simulink model "SimulationANTSMC"  (R2020b)
(part 15 of 18)

                                                                                                                                                                                                                                                                                                                                                                                                                                                                                                                                                                                                                                                                                                                                                                                                                                                                                                                                                                                                                                                                                                                                                                                                                                                                                                                                                                                                                                                                                                                                                                                                                                                                                                                                                                                                                                                                                                                                                                                                                                                                                                                                                                                                                                                                                                                                                                                                                                                                                                                                                                                                                                                                                                                                                                                                                                                                                                                                                                                                                                                                                                                                                                                                                                                                                                                                                                                                                                                                                                                                                                                                                                                                                                                                                                                                                                                                                                                                                                                                                                                                                                                                                                                                                                                                                                                                                                                                                                                                                                                                                                                                                                                                                                                                                                                                                                                                                                                                                                                                                                                                                                                                                                                                                                                                                                                                                                                                                                                                                                                                                                                                                                                                                                                                                                                                                                                                                                                                                                                                                                                                                                                                                                                                                                                                                                                                                                                                                                                                                                                                                                                                                                                                                                                                                                                                                                                                                                                                                                                                                                                                                                                                                                                                                                                                                                                                                                                                                                                                                                                                                                                                                                                                                                                                                                                                                                                                                                                                                                                                                                                                                                                                                                                                                                                                                                                                                                                                                                                                                                                                                                                                                                                                                                                                                                                                                                                                                                                                                                                                                                                                                                                                                                                                                                                                                                                                                                                                                                                                                                                                                                                                                                                                                                                                                                                                                                                                                                                                                                                                                                                                                                                                                                                                                                                                                                                                                                                                                                                                                                                                                                                                                                                                                                                                                                                                                                                                                                                                                                                                                                                                                                                                                                                                                                                                                                                                                                                                                                                                                                                                                                                                                                                                                                                                                                                                                                                                                                                                                                                                                                                                                                                                                                                                                                                                                                                                                                                                                                                                                                                                                                                                                                                                                                                                                                                                                                                                                                                                                                                                                                                                                                                                                                                                                                                                                                                                                                                                                                                                                                                                                                                                                                                                                                                                                                                                                                                                                                                                                                                                                                                                                                                                                                                                                                                                                                                                                                                                                                                                                                                                                                                                                                                                                                                                                                                                                                                                                                                                                                                                                                                                                                                                                                                                                                                                                                                                                                                                                                                                                                                                                                                                                                                                                                                                                                                                                                                                                                                                                                                                                                                                                                                                                                                                                                                                                                                                                                                                                                                                                                                                                                                                                                                                                                                                                                                                                                                                                                                                                                                                                                                                                                                                                                                                                                                                                                                                                                                                                                                                                                                                                                                                                                                                                                                                                                                                                                                                                                                                                                                                                                                                                                                                                                                                                                                                                                                                                                                                                                                                                                                                                                                                                                                                                                                                                                                                                                                                                                                                                                                                                                                                                                                                                                                                                                                                                                                                                                                                                                                                                                                                                                                                                                                                                                                                                                                                                                                                                                                                                                                                                                                                                                                                                                                                                                                                                                                                                                                                                                                                                                                                                                                                                                                                                                                                                                                                                                                                                                                                                                                                                                                                                                                                                                                                                                                                                                                                                                                                                                                                                                                                                                                                                                                                                                                                                                                                                                                                                                                                                                                                                                                                                                                                                                                                                                                                                                                                                                                                                                                                                                                                                                                                                                                                                                                                                                                                                                                                                                                                                                                                                                                                                                                                                                                                                                                                                                                                                                                                                                                                                                                                                                                                                                                                                                                                                                                                                                                                                                                                                                                                                                                                                                                                                                                                                                                                                                                                                                                                                                                                                                                                                                                                                                                                                                                                                                                                                                                                                                                                                                                                                                                                                                                                                                                                                                                                                                                                                                                                                                                                                                                                                                                                                                                                                                                                                                                                                                                                                                                                                                                                                                                                                                                                                                                                                                                                                                                                                                                                                                                                                                                                                                                                                                                                                                                                                                                                                                                                                                                                                                                                                                                                                                                                                                                                                                                                                                                                                                                                                                                                                                                                                                                                                                                                                                                                                                                                                                                                                                                                                                                                                                                                                                                                                                                                                                                                                                                                                                                                                                                                                                                                                                                                                                                                                                                                                                                                                                                                                                                                                                                                                                                                                                                                                                                                                                                                                                                                                                                                                                                                                                                                                                                                                                                                                                                                                                                                                                                                                                                                                                                                                                                                                                                                                                                                                                                                                                                                                                                                                                                                                                                                                                                                                                                                                                                                                                                                                                                                                                                                                                                                                                                                                                                                                                                                                                                                                                                                                                                                                                                                                                                                                                                                                                                                                                                                                                                                                                                                                                                                                                                                                                                                                                                                                                                                                                                                                                                                                                                                                                                                                                                                                                                                                                                                                                                                                                                                                                                                                                                                                                                                                                                                                                                                                                                                                                                                                                                                                                                                                                                                                                                                                                                                                                                                                                                                                                                                                                                                                                                                                                                                                                                                                                                                                                                                                                                                                                                                                                                                                                                                                                                                                                                                                                                                                                                                                                                                                                                                                                                                                                                                                                                                                                                                                                                                                                                                                                                                                                                                                                                                                                                                                                                                                                                                                                                                                                                                                                                                                                                                                                                                                                                                                                                                                                                                                                                                                                                                                                                                                                                                                                                                                                                                                                                                                                                                                                                                                                                                                                                                                                                                                                                                                                                                                                                                                                                                                                                                                                                                                                                                                                                                                                                                                                                                                                                                                                                                                                                                                                                                                                                                                                                                                                                                                                                                                                                                                                                                                                                                                                                                                                                                                                                                                                                                                                                                                                                                                                                                                                                                                                                                                                                                                                                                                                                                                                                                                                                                                                                                                                                                                                                                                                                                                                                                                                                                                                                                                                                                                                                                                                                                                                                                                                                                                                                                                                                                                                                                                                                                                                                                                                                                                                                                                                                                                                                                                                                                                                                                                                                                                                                                                                                                                                                                                                                                                                                                                                                                                                                                                                                                                                                                                                                                                                                                                                                                                                                                                                                                                                                                                                                                                                                                                                                                                                                                                                                                                                                                                                                                                                                                                                                                                                                                                                                                                                                                                                                                                                                                                                                                                                                                                                                                                                                                                                                                                                                                                                                                                                                                                                                                                                                                                                                                                                                                                                                                                                                                                                                                                                                                                                                                                                                                                                                                                                                                                                                                                                                                                                                                                                                                                                                                                                                                                                                                                                                                                                                                                                                                                                                                                                                                                                                                                                                                                                                                                                                                                                                                                                                                                                                                                                                                                                                                                                                                                                                                                                                                                                                                                                                                                                                                                                                                                                                                                                                                                                                                                                                                                                                                                                                                                                                                                                                                                                                                                                                                                                                                                                                                                                                                                                                                                                                                                                                                                                                                                                                                                                                                                                                                                                                                                                                                                                                                                                                                                                                                                                                                                                                                                                                                                                                                                                                                                                                                                                                                                                                                                                                                                                                                                                                                                                                                                                                                                                                                                                                                                                                                                                                                                                                                                                                                                                                                                                                                                                                                                                                                                                                                                                                                                                                                                                                                                                                                                                                                                                                                                                                                                                                                                                                                                                                                                                                                                                                                                                                                                                                                                                                                                                                                                                                                                                                                                                                                                                                                                                                                                                                                                                                                                                                                                                                                                                                                                                                                                                                                                                                                                                                                                                                                                                                                                                                                                                                                                                                                                                                                                                                                                                                                                                                                                                                                                                                                                                                                                                                                                                                                                                                                                                                                                                                                                                                                                                                                                                                                                                                                                                                                                                                                                                                                                                                                                                                                                                                                                                                                                                                                                                                                                                                                                                                                                                                                                                                                                                                                                                                                                                                                                                                                                                                                                                                                                                                                                                                                                                                                                                                                                                                                                                                                                                                                                                                                                                                                                                                                                                                                                                                                                                                                                                                                                                                                                                                                                                                                                                                                                                                                                                                                                                                                                                                                                                                                                                                                                                                                                                                                                                                                                                                                                                                                                                                                                                                                                                                                                                                                                                                                                                                                                                                                                                                                                                                                                                                                                                                                                                                                                                                                                                                                                                                                                                                                                                                                                                                                                                                                                                                                                                                                                                                                                                                                                                                                                                                                                                                                                                                                                                                                                                                                                                                                                                                                                                                                                                                                                                                                                                                                                                                                                                                                                                                                                                                                                                                                                                                                                                                                                                                                                                                                                                                                                                                                                                                                                                                                                                                                                                                                                                                                                                                                                                                                                                                                                                                                                                                                                                                                                                                                                                                                                                                                                                                                                                                                                                                                                                                                                                                                                                                                                                                                                                                                                                                                                                                                                                                                                                                                                                                                                                                                                                                                                                                                                                                                                                                                                                                                                                                                                                                                                                                                                                                                                                                                                                                                                                                                                                                                                                                                                                                                                                                                                                                                                                                                                                                                                                                                                                                                                                                                                                                                                                                                                                                                                                                                                                                                                                                                                                                                                                                                                                                                                                                                                                                                                                                                                                                                                                                                                                                                                                                                                                                                                                                                                                                                                                                                                                                                                                                                                                                                                                                                                                                                                                                                                                                                                                                                                                                                                                                                                                                                                                                                                                                                                                                                                                                                                                                                                                                                                                                                                                                                                                                                                                                                                                                                                                                                                                                                                                                                                                                                                                                                                                                                                                                                                                                                                                                                                                                                                                                                                                                                                                                                                                                                                                                                                                                                                                                                                                                                                                                                                                                                                                                                                                                                                                                                                                                                                                                                                                                                                                                                                                                                                                                                                                                                                                                                                                                                                                                                                                                                                                                                                                                                                                                                                                                                                                                                                                                                                                                                                                                                                                                                                                                                                                                                                                                                                                                                                                                                                                                                                                                                                                                                                                                                                                                                                                                                                                                                                                                                                                                                                                                                                                                                                                                                                                                                                                                                                                                                                                                                                                                                                                                                                                                                                                                                                                                                                                                                                                                                                                                                                                                                                                                                                                                                                                                                                                                                                                                                                                                                                                                                                                                                                                                                                                                                                                                                                                                                                                                                                                                                                                                                                                                                                                                                                                                                                                                                                                                                                                                                                                                                                                                                                                                                                                                                                                                                                                                                                                                                                                                                                                                                                                                                                                                                                                                                                                                                                                                                                                                                                                                                                                                                                                                                                                                                                                                                                                                                                                                                                                                                                                                                                                                                                                                                                                                                                                                                                                                                                                                                                                                                                                                                                                                                                                                                                                                                                                                                                                                                                                                                                                                                                                                                                                                                                                                                                                                                                                                                                                                                                                                                                                                                                                                                                                                                                                                                                                                                                                                                                                                                                                                                                                                                                                                                                                                                                                                                                                                                                                                                                                                                                                                                                                0.02*thetadot1^2*sin(2*theta6) - 0.02*thetadot4^2*sin(2*theta6) + 0.02*thetadot5^2*sin(2*theta6) + 0.3*thetadot1^2*sin(theta5)*sin(theta6) + 0.3*thetadot2^2*sin(theta5)*sin(theta6) + 0.3*thetadot3^2*sin(theta5)*sin(theta6) - 0.0001*thetadot4*thetadot5*sin(theta5) + 0.0801*thetadot2*thetadot4*cos(theta4)*sin(theta5) + 0.0001*thetadot2*thetadot5*cos(theta5)*sin(theta4) + 0.0801*thetadot3*thetadot4*cos(theta4)*sin(theta5) + 0.0001*thetadot3*thetadot5*cos(theta5)*sin(theta4) + 0.6*thetadot2*thetadot3*sin(theta5)*sin(theta6) + 0.56*thetadot2*thetadot4*sin(theta4)*sin(theta6) + 0.56*thetadot3*thetadot4*sin(theta4)*sin(theta6) - 0.08*thetadot1^2*cos(theta2)^2*cos(theta6)*sin(theta6) - 0.08*thetadot1^2*cos(theta3)^2*cos(theta6)*sin(theta6) - 0.04*thetadot1^2*cos(theta4)^2*cos(theta6)*sin(theta6) + 0.04*thetadot2^2*cos(theta4)^2*cos(theta6)*sin(theta6) - 0.04*thetadot2^2*cos(theta5)^2*cos(theta6)*sin(theta6) + 0.04*thetadot3^2*cos(theta4)^2*cos(theta6)*sin(theta6) - 0.04*thetadot3^2*cos(theta5)^2*cos(theta6)*sin(theta6) + 0.04*thetadot4^2*cos(theta5)^2*cos(theta6)*sin(theta6) - 0.3*thetadot1^2*cos(theta2)^2*sin(theta5)*sin(theta6) - 0.3*thetadot1^2*cos(theta3)^2*sin(theta5)*sin(theta6) - 0.08*thetadot4*thetadot5*cos(theta6)^2*sin(theta5) + 0.04*thetadot1^2*cos(theta4)*cos(theta5)*sin(theta4) - 0.04*thetadot2^2*cos(theta4)*cos(theta5)*sin(theta4) - 0.04*thetadot3^2*cos(theta4)*cos(theta5)*sin(theta4) + 0.12*thetadot2^2*cos(theta6)*sin(theta3)*sin(theta4) + 0.12*thetadot2^2*cos(theta3)*sin(theta5)*sin(theta6) - 0.28*thetadot2^2*cos(theta5)*sin(theta5)*sin(theta6) - 0.28*thetadot3^2*cos(theta5)*sin(theta5)*sin(theta6) + 0.28*thetadot4^2*cos(theta5)*sin(theta5)*sin(theta6) + 0.56*thetadot4*thetadot5*cos(theta5)*cos(theta6) - 0.04*thetadot1^2*cos(theta2)^2*cos(theta4)*cos(theta5)*sin(theta4) - 0.04*thetadot1^2*cos(theta3)^2*cos(theta4)*cos(theta5)*sin(theta4) - 0.08*thetadot1^2*cos(theta4)*cos(theta5)*cos(theta6)^2*sin(theta4) + 0.08*thetadot2^2*cos(theta4)*cos(theta5)*cos(theta6)^2*sin(theta4) + 0.08*thetadot3^2*cos(theta4)*cos(theta5)*cos(theta6)^2*sin(theta4) + 0.12*thetadot1^2*cos(theta2)^2*cos(theta6)*sin(theta3)*sin(theta4) + 0.12*thetadot1^2*cos(theta2)^2*cos(theta3)*sin(theta5)*sin(theta6) + 0.28*thetadot1^2*cos(theta2)^2*cos(theta5)*sin(theta5)*sin(theta6) + 0.28*thetadot1^2*cos(theta3)^2*cos(theta5)*sin(theta5)*sin(theta6) - 0.28*thetadot1^2*cos(theta4)^2*cos(theta5)*sin(theta5)*sin(theta6) + 0.28*thetadot2^2*cos(theta4)^2*cos(theta5)*sin(theta5)*sin(theta6) + 0.28*thetadot3^2*cos(theta4)^2*cos(theta5)*sin(theta5)*sin(theta6) + 0.08*thetadot2*thetadot3*cos(theta4)^2*cos(theta6)*sin(theta6) - 0.08*thetadot2*thetadot4*cos(theta4)*cos(theta6)^2*sin(theta5) - 0.08*thetadot2*thetadot3*cos(theta5)^2*cos(theta6)*sin(theta6) + 0.08*thetadot2*thetadot5*cos(theta5)*cos(theta6)^2*sin(theta4) - 0.08*thetadot3*thetadot4*cos(theta4)*cos(theta6)^2*sin(theta5) + 0.08*thetadot3*thetadot5*cos(theta5)*cos(theta6)^2*sin(theta4) - 0.56*thetadot2*thetadot4*cos(theta5)^2*sin(theta4)*sin(theta6) - 0.56*thetadot3*thetadot4*cos(theta5)^2*sin(theta4)*sin(theta6) + 0.16*thetadot1^2*cos(theta2)^2*cos(theta3)^2*cos(theta6)*sin(theta6) + 0.04*thetadot1^2*cos(theta2)^2*cos(theta4)^2*cos(theta6)*sin(theta6) + 0.04*thetadot1^2*cos(theta2)^2*cos(theta5)^2*cos(theta6)*sin(theta6) + 0.04*thetadot1^2*cos(theta3)^2*cos(theta4)^2*cos(theta6)*sin(theta6) + 0.04*thetadot1^2*cos(theta3)^2*cos(theta5)^2*cos(theta6)*sin(theta6) - 0.04*thetadot1^2*cos(theta4)^2*cos(theta5)^2*cos(theta6)*sin(theta6) + 0.04*thetadot2^2*cos(theta4)^2*cos(theta5)^2*cos(theta6)*sin(theta6) + 0.04*thetadot3^2*cos(theta4)^2*cos(theta5)^2*cos(theta6)*sin(theta6) + 0.6*thetadot1^2*cos(theta2)^2*cos(theta3)^2*sin(theta5)*sin(theta6) - 0.28*thetadot1^2*cos(theta2)*cos(theta4)*sin(theta2)*sin(theta6) - 0.3*thetadot1^2*cos(theta2)*cos(theta6)*sin(theta2)*sin(theta4) - 0.28*thetadot1^2*cos(theta3)*cos(theta4)*sin(theta3)*sin(theta6) - 0.3*thetadot1^2*cos(theta3)*cos(theta6)*sin(theta3)*sin(theta4) - 0.28*thetadot1^2*cos(theta4)*cos(theta6)*sin(theta4)*sin(theta5) + 0.12*thetadot2^2*cos(theta4)*cos(theta5)*sin(theta3)*sin(theta6) + 0.28*thetadot2^2*cos(theta4)*cos(theta6)*sin(theta4)*sin(theta5) + 0.28*thetadot3^2*cos(theta4)*cos(theta6)*sin(theta4)*sin(theta5) + 0.04*thetadot1^2*cos(theta2)*sin(theta2)*sin(theta4)*sin(theta5) + 0.04*thetadot1^2*cos(theta3)*sin(theta3)*sin(theta4)*sin(theta5) + 0.0801*thetadot1*thetadot2*cos(theta2)*cos(theta3)*cos(theta5) + 0.0801*thetadot1*thetadot3*cos(theta2)*cos(theta3)*cos(theta5) - 0.24*thetadot1*thetadot2*cos(theta4)*cos(theta6)*sin(theta2) - 0.08*thetadot2*thetadot3*cos(theta4)*cos(theta5)*sin(theta4) + 0.08*thetadot2*thetadot5*cos(theta4)*cos(theta6)*sin(theta6) + 0.08*thetadot3*thetadot5*cos(theta4)*cos(theta6)*sin(theta6) - 0.0801*thetadot1*thetadot2*cos(theta5)*sin(theta2)*sin(theta3) - 0.0801*thetadot1*thetadot3*cos(theta5)*sin(theta2)*sin(theta3) - 0.0001*thetadot1*thetadot5*cos(theta2)*sin(theta3)*sin(theta5) - 0.0001*thetadot1*thetadot5*cos(theta3)*sin(theta2)*sin(theta5) - 0.56*thetadot2*thetadot3*cos(theta5)*sin(theta5)*sin(theta6) + 0.56*thetadot2*thetadot5*cos(theta6)*sin(theta4)*sin(theta5) + 0.56*thetadot3*thetadot5*cos(theta6)*sin(theta4)*sin(theta5) - 0.08*thetadot1*thetadot2*cos(theta2)*cos(theta3)*cos(theta4)^2*cos(theta5) - 0.08*thetadot1*thetadot3*cos(theta2)*cos(theta3)*cos(theta4)^2*cos(theta5) - 0.08*thetadot1*thetadot2*cos(theta2)*cos(theta3)*cos(theta5)*cos(theta6)^2 - 0.08*thetadot1*thetadot3*cos(theta2)*cos(theta3)*cos(theta5)*cos(theta6)^2 + 0.16*thetadot2*thetadot3*cos(theta4)*cos(theta5)*cos(theta6)^2*sin(theta4) + 0.08*thetadot1*thetadot2*cos(theta4)^2*cos(theta5)*sin(theta2)*sin(theta3) + 0.08*thetadot1*thetadot3*cos(theta4)^2*cos(theta5)*sin(theta2)*sin(theta3) + 0.08*thetadot1*thetadot2*cos(theta5)*cos(theta6)^2*sin(theta2)*sin(theta3) + 0.08*thetadot1*thetadot3*cos(theta5)*cos(theta6)^2*sin(theta2)*sin(theta3) - 0.08*thetadot1*thetadot5*cos(theta2)*cos(theta6)^2*sin(theta3)*sin(theta5) - 0.08*thetadot1*thetadot5*cos(theta3)*cos(theta6)^2*sin(theta2)*sin(theta5) + 0.56*thetadot2*thetadot3*cos(theta4)^2*cos(theta5)*sin(theta5)*sin(theta6) + 0.08*thetadot1^2*cos(theta2)^2*cos(theta3)^2*cos(theta4)*cos(theta5)*sin(theta4) + 0.08*thetadot1^2*cos(theta2)^2*cos(theta4)*cos(theta5)*cos(theta6)^2*sin(theta4) + 0.08*thetadot1^2*cos(theta3)^2*cos(theta4)*cos(theta5)*cos(theta6)^2*sin(theta4) - 0.56*thetadot1^2*cos(theta2)^2*cos(theta3)^2*cos(theta5)*sin(theta5)*sin(theta6) + 0.28*thetadot1^2*cos(theta2)^2*cos(theta4)^2*cos(theta5)*sin(theta5)*sin(theta6) + 0.28*thetadot1^2*cos(theta3)^2*cos(theta4)^2*cos(theta5)*sin(theta5)*sin(theta6) + 0.08*thetadot2*thetadot3*cos(theta4)^2*cos(theta5)^2*cos(theta6)*sin(theta6) + 0.12*thetadot1^2*cos(theta2)*cos(theta3)*cos(theta6)*sin(theta2)*sin(theta4) - 0.3*thetadot1^2*cos(theta2)*cos(theta4)*cos(theta5)*sin(theta2)*sin(theta6) + 0.28*thetadot1^2*cos(theta2)*cos(theta5)*cos(theta6)*sin(theta2)*sin(theta4) - 0.3*thetadot1^2*cos(theta3)*cos(theta4)*cos(theta5)*sin(theta3)*sin(theta6) + 0.28*thetadot1^2*cos(theta3)*cos(theta5)*cos(theta6)*sin(theta3)*sin(theta4) - 0.08*thetadot1^2*cos(theta2)^2*cos(theta3)^2*cos(theta4)^2*cos(theta6)*sin(theta6) - 0.08*thetadot1^2*cos(theta2)^2*cos(theta3)^2*cos(theta5)^2*cos(theta6)*sin(theta6) + 0.04*thetadot1^2*cos(theta2)^2*cos(theta4)^2*cos(theta5)^2*cos(theta6)*sin(theta6) + 0.04*thetadot1^2*cos(theta3)^2*cos(theta4)^2*cos(theta5)^2*cos(theta6)*sin(theta6) + 0.0001*thetadot1*thetadot5*cos(theta2)*cos(theta3)*cos(theta4)*cos(theta5) - 0.12*thetadot1^2*cos(theta2)*sin(theta2)*sin(theta3)*sin(theta5)*sin(theta6) - 0.6*thetadot1*thetadot2*cos(theta2)*cos(theta4)*cos(theta6)*sin(theta3) - 0.6*thetadot1*thetadot2*cos(theta3)*cos(theta4)*cos(theta6)*sin(theta2) - 0.6*thetadot1*thetadot3*cos(theta2)*cos(theta4)*cos(theta6)*sin(theta3) - 0.6*thetadot1*thetadot3*cos(theta3)*cos(theta4)*cos(theta6)*sin(theta2) + 0.56*thetadot1*thetadot4*cos(theta2)*cos(theta3)*cos(theta4)*sin(theta6) + 0.56*thetadot1*thetadot5*cos(theta2)*cos(theta5)*cos(theta6)*sin(theta3) + 0.56*thetadot1*thetadot5*cos(theta3)*cos(theta5)*cos(theta6)*sin(theta2) - 0.0001*thetadot1*thetadot2*cos(theta2)*cos(theta4)*sin(theta3)*sin(theta5) - 0.0001*thetadot1*thetadot2*cos(theta3)*cos(theta4)*sin(theta2)*sin(theta5) - 0.0001*thetadot1*thetadot3*cos(theta2)*cos(theta4)*sin(theta3)*sin(theta5) - 0.0001*thetadot1*thetadot3*cos(theta3)*cos(theta4)*sin(theta2)*sin(theta5) - 0.0801*thetadot1*thetadot4*cos(theta2)*cos(theta3)*sin(theta4)*sin(theta5) + 4.4200467277063457510618654694995e-35*thetadot1*thetadot4*cos(theta2)*cos(theta6)*sin(theta3)*sin(theta4) + 4.4200467277063457510618654694995e-35*thetadot1*thetadot4*cos(theta3)*cos(theta6)*sin(theta2)*sin(theta4) - 0.0001*thetadot1*thetadot5*cos(theta4)*cos(theta5)*sin(theta2)*sin(theta3) - 0.08*thetadot1*thetadot4*cos(theta2)*cos(theta6)*sin(theta3)*sin(theta6) - 0.08*thetadot1*thetadot4*cos(theta3)*cos(theta6)*sin(theta2)*sin(theta6) + 0.56*thetadot2*thetadot3*cos(theta4)*cos(theta6)*sin(theta4)*sin(theta5) + 0.24*thetadot1*thetadot2*cos(theta5)*sin(theta2)*sin(theta4)*sin(theta6) - 0.56*thetadot1*thetadot4*cos(theta4)*sin(theta2)*sin(theta3)*sin(theta6) + 0.0801*thetadot1*thetadot4*sin(theta2)*sin(theta3)*sin(theta4)*sin(theta5) + 0.56*thetadot1^2*cos(theta2)*cos(theta3)^2*cos(theta4)*sin(theta2)*sin(theta6) + 0.6*thetadot1^2*cos(theta2)*cos(theta3)^2*cos(theta6)*sin(theta2)*sin(theta4) + 0.56*thetadot1^2*cos(theta2)^2*cos(theta3)*cos(theta4)*sin(theta3)*sin(theta6) + 0.6*thetadot1^2*cos(theta2)^2*cos(theta3)*cos(theta6)*sin(theta3)*sin(theta4) + 0.56*thetadot1^2*cos(theta2)*cos(theta4)*cos(theta5)^2*sin(theta2)*sin(theta6) + 0.12*thetadot1^2*cos(theta2)^2*cos(theta4)*cos(theta5)*sin(theta3)*sin(theta6) + 0.56*thetadot1^2*cos(theta3)*cos(theta4)*cos(theta5)^2*sin(theta3)*sin(theta6) + 0.28*thetadot1^2*cos(theta2)^2*cos(theta4)*cos(theta6)*sin(theta4)*sin(theta5) + 0.28*thetadot1^2*cos(theta3)^2*cos(theta4)*cos(theta6)*sin(theta4)*sin(theta5) - 0.08*thetadot1^2*cos(theta2)*cos(theta3)^2*sin(theta2)*sin(theta4)*sin(theta5) - 0.08*thetadot1^2*cos(theta2)^2*cos(theta3)*sin(theta3)*sin(theta4)*sin(theta5) - 0.08*thetadot1^2*cos(theta2)*cos(theta6)^2*sin(theta2)*sin(theta4)*sin(theta5) - 0.08*thetadot1^2*cos(theta3)*cos(theta6)^2*sin(theta3)*sin(theta4)*sin(theta5) - 0.56*thetadot1*thetadot2*cos(theta2)*cos(theta5)^2*sin(theta3)*sin(theta4)*sin(theta6) - 0.56*thetadot1*thetadot2*cos(theta3)*cos(theta5)^2*sin(theta2)*sin(theta4)*sin(theta6) - 0.56*thetadot1*thetadot2*cos(theta4)^2*cos(theta6)*sin(theta2)*sin(theta3)*sin(theta5) - 0.56*thetadot1*thetadot3*cos(theta2)*cos(theta5)^2*sin(theta3)*sin(theta4)*sin(theta6) - 0.56*thetadot1*thetadot3*cos(theta3)*cos(theta5)^2*sin(theta2)*sin(theta4)*sin(theta6) - 0.56*thetadot1*thetadot3*cos(theta4)^2*cos(theta6)*sin(theta2)*sin(theta3)*sin(theta5) + 0.56*thetadot1*thetadot4*cos(theta4)*cos(theta5)^2*sin(theta2)*sin(theta3)*sin(theta6) - 0.08*thetadot1*thetadot4*cos(theta6)^2*sin(theta2)*sin(theta3)*sin(theta4)*sin(theta5) - 1.12*thetadot1^2*cos(theta2)*cos(theta3)^2*cos(theta4)*cos(theta5)^2*sin(theta2)*sin(theta6) - 1.12*thetadot1^2*cos(theta2)^2*cos(theta3)*cos(theta4)*cos(theta5)^2*sin(theta3)*sin(theta6) - 0.56*thetadot1^2*cos(theta2)^2*cos(theta3)^2*cos(theta4)*cos(theta6)*sin(theta4)*sin(theta5) + 0.16*thetadot1^2*cos(theta2)*cos(theta3)^2*cos(theta6)^2*sin(theta2)*sin(theta4)*sin(theta5) + 0.16*thetadot1^2*cos(theta2)^2*cos(theta3)*cos(theta6)^2*sin(theta3)*sin(theta4)*sin(theta5) + 0.16*thetadot1*thetadot2*cos(theta2)*cos(theta3)*cos(theta4)^2*cos(theta5)*cos(theta6)^2 + 0.16*thetadot1*thetadot3*cos(theta2)*cos(theta3)*cos(theta4)^2*cos(theta5)*cos(theta6)^2 - 0.16*thetadot1*thetadot2*cos(theta4)^2*cos(theta5)*cos(theta6)^2*sin(theta2)*sin(theta3) - 0.16*thetadot1*thetadot3*cos(theta4)^2*cos(theta5)*cos(theta6)^2*sin(theta2)*sin(theta3) + 0.12*thetadot1^2*cos(theta2)*cos(theta3)*cos(theta4)*cos(theta5)*sin(theta2)*sin(theta6) - 0.16*thetadot1^2*cos(theta2)^2*cos(theta3)^2*cos(theta4)*cos(theta5)*cos(theta6)^2*sin(theta4) - 0.16*thetadot1^2*cos(theta2)*cos(theta3)*cos(theta6)*sin(theta2)*sin(theta3)*sin(theta6) - 0.56*thetadot1^2*cos(theta2)^2*cos(theta3)^2*cos(theta4)^2*cos(theta5)*sin(theta5)*sin(theta6) - 0.6*thetadot1^2*cos(theta2)*cos(theta3)*sin(theta2)*sin(theta3)*sin(theta5)*sin(theta6) + 0.56*thetadot1*thetadot2*cos(theta2)*cos(theta4)*cos(theta5)*cos(theta6)*sin(theta3) + 0.56*thetadot1*thetadot2*cos(theta3)*cos(theta4)*cos(theta5)*cos(theta6)*sin(theta2) + 0.56*thetadot1*thetadot3*cos(theta2)*cos(theta4)*cos(theta5)*cos(theta6)*sin(theta3) + 0.56*thetadot1*thetadot3*cos(theta3)*cos(theta4)*cos(theta5)*cos(theta6)*sin(theta2) + 1.041784545864672835129637359261e-36*thetadot1*thetadot4*cos(theta2)*cos(theta3)*cos(theta4)*cos(theta5)*sin(theta6) + 0.56*thetadot1*thetadot5*cos(theta2)*cos(theta3)*cos(theta4)*cos(theta6)*sin(theta5) + 4.4200467277063457510618654694995e-35*thetadot1*thetadot4*cos(theta2)*cos(theta4)*cos(theta5)*sin(theta3)*sin(theta6) + 4.4200467277063457510618654694995e-35*thetadot1*thetadot4*cos(theta3)*cos(theta4)*cos(theta5)*sin(theta2)*sin(theta6) - 0.08*thetadot1*thetadot5*cos(theta2)*cos(theta3)*cos(theta6)*sin(theta4)*sin(theta6) + 0.6*thetadot1*thetadot2*cos(theta2)*cos(theta5)*sin(theta3)*sin(theta4)*sin(theta6) + 0.6*thetadot1*thetadot2*cos(theta3)*cos(theta5)*sin(theta2)*sin(theta4)*sin(theta6) + 0.6*thetadot1*thetadot3*cos(theta2)*cos(theta5)*sin(theta3)*sin(theta4)*sin(theta6) + 0.6*thetadot1*thetadot3*cos(theta3)*cos(theta5)*sin(theta2)*sin(theta4)*sin(theta6) - 1.041784545864672835129637359261e-36*thetadot1*thetadot4*cos(theta4)*cos(theta5)*sin(theta2)*sin(theta3)*sin(theta6) + 0.56*thetadot1*thetadot4*cos(theta2)*cos(theta5)*sin(theta3)*sin(theta5)*sin(theta6) + 0.56*thetadot1*thetadot4*cos(theta3)*cos(theta5)*sin(theta2)*sin(theta5)*sin(theta6) - 0.56*thetadot1*thetadot5*cos(theta4)*cos(theta6)*sin(theta2)*sin(theta3)*sin(theta5) + 0.08*thetadot2*thetadot4*cos(theta5)*cos(theta6)*sin(theta4)*sin(theta5)*sin(theta6) + 0.08*thetadot3*thetadot4*cos(theta5)*cos(theta6)*sin(theta4)*sin(theta5)*sin(theta6) + 0.08*thetadot1*thetadot5*cos(theta6)*sin(theta2)*sin(theta3)*sin(theta4)*sin(theta6) + 0.6*thetadot1^2*cos(theta2)*cos(theta3)^2*cos(theta4)*cos(theta5)*sin(theta2)*sin(theta6) - 0.56*thetadot1^2*cos(theta2)*cos(theta3)^2*cos(theta5)*cos(theta6)*sin(theta2)*sin(theta4) + 0.6*thetadot1^2*cos(theta2)^2*cos(theta3)*cos(theta4)*cos(theta5)*sin(theta3)*sin(theta6) - 0.56*thetadot1^2*cos(theta2)^2*cos(theta3)*cos(theta5)*cos(theta6)*sin(theta3)*sin(theta4) - 0.08*thetadot1^2*cos(theta2)^2*cos(theta3)^2*cos(theta4)^2*cos(theta5)^2*cos(theta6)*sin(theta6) + 0.08*thetadot1*thetadot5*cos(theta2)*cos(theta3)*cos(theta4)*cos(theta5)*cos(theta6)^2 + 0.56*thetadot1*thetadot2*cos(theta2)*cos(theta3)*cos(theta4)^2*cos(theta6)*sin(theta5) + 0.56*thetadot1*thetadot3*cos(theta2)*cos(theta3)*cos(theta4)^2*cos(theta6)*sin(theta5) - 0.56*thetadot1*thetadot4*cos(theta2)*cos(theta3)*cos(theta4)*cos(theta5)^2*sin(theta6) - 0.08*thetadot1*thetadot2*cos(theta2)*cos(theta4)*cos(theta6)^2*sin(theta3)*sin(theta5) - 0.08*thetadot1*thetadot2*cos(theta3)*cos(theta4)*cos(theta6)^2*sin(theta2)*sin(theta5) - 0.08*thetadot1*thetadot3*cos(theta2)*cos(theta4)*cos(theta6)^2*sin(theta3)*sin(theta5) - 0.08*thetadot1*thetadot3*cos(theta3)*cos(theta4)*cos(theta6)^2*sin(theta2)*sin(theta5) + 0.08*thetadot1*thetadot4*cos(theta2)*cos(theta3)*cos(theta6)^2*sin(theta4)*sin(theta5) - 0.08*thetadot1*thetadot5*cos(theta4)*cos(theta5)*cos(theta6)^2*sin(theta2)*sin(theta3) + 0.08*thetadot1*thetadot4*cos(theta2)*cos(theta5)^2*cos(theta6)*sin(theta3)*sin(theta6) + 0.08*thetadot1*thetadot4*cos(theta3)*cos(theta5)^2*cos(theta6)*sin(theta2)*sin(theta6) - 0.08*thetadot1^2*cos(theta2)*cos(theta3)*cos(theta4)*cos(theta5)*sin(theta2)*sin(theta3)*sin(theta4) - 0.08*thetadot1^2*cos(theta2)*cos(theta4)*cos(theta5)*cos(theta6)*sin(theta2)*sin(theta5)*sin(theta6) - 0.08*thetadot1^2*cos(theta3)*cos(theta4)*cos(theta5)*cos(theta6)*sin(theta3)*sin(theta5)*sin(theta6) + 0.56*thetadot1^2*cos(theta2)*cos(theta3)*cos(theta5)*sin(theta2)*sin(theta3)*sin(theta5)*sin(theta6) - 0.08*thetadot1*thetadot2*cos(theta2)*cos(theta3)*cos(theta4)*cos(theta6)*sin(theta4)*sin(theta6) - 0.08*thetadot1*thetadot3*cos(theta2)*cos(theta3)*cos(theta4)*cos(theta6)*sin(theta4)*sin(theta6) + 0.08*thetadot1*thetadot2*cos(theta4)*cos(theta6)*sin(theta2)*sin(theta3)*sin(theta4)*sin(theta6) + 0.08*thetadot1*thetadot3*cos(theta4)*cos(theta6)*sin(theta2)*sin(theta3)*sin(theta4)*sin(theta6) + 0.08*thetadot1^2*cos(theta2)*cos(theta3)*cos(theta4)^2*cos(theta6)*sin(theta2)*sin(theta3)*sin(theta6) + 0.08*thetadot1^2*cos(theta2)*cos(theta3)*cos(theta5)^2*cos(theta6)*sin(theta2)*sin(theta3)*sin(theta6) + 0.56*thetadot1^2*cos(theta2)*cos(theta3)*cos(theta4)*cos(theta6)*sin(theta2)*sin(theta3)*sin(theta4)*sin(theta5) + 0.08*thetadot1*thetadot4*cos(theta2)*cos(theta3)*cos(theta4)*cos(theta5)*cos(theta6)*sin(theta5)*sin(theta6) - 0.56*thetadot1*thetadot2*cos(theta2)*cos(theta3)*cos(theta4)*cos(theta5)*sin(theta4)*sin(theta5)*sin(theta6) - 0.56*thetadot1*thetadot3*cos(theta2)*cos(theta3)*cos(theta4)*cos(theta5)*sin(theta4)*sin(theta5)*sin(theta6) + 0.08*thetadot1*thetadot2*cos(theta2)*cos(theta5)*cos(theta6)*sin(theta3)*sin(theta4)*sin(theta5)*sin(theta6) + 0.08*thetadot1*thetadot2*cos(theta3)*cos(theta5)*cos(theta6)*sin(theta2)*sin(theta4)*sin(theta5)*sin(theta6) + 0.08*thetadot1*thetadot3*cos(theta2)*cos(theta5)*cos(theta6)*sin(theta3)*sin(theta4)*sin(theta5)*sin(theta6) + 0.08*thetadot1*thetadot3*cos(theta3)*cos(theta5)*cos(theta6)*sin(theta2)*sin(theta4)*sin(theta5)*sin(theta6) - 0.08*thetadot1*thetadot4*cos(theta4)*cos(theta5)*cos(theta6)*sin(theta2)*sin(theta3)*sin(theta5)*sin(theta6) + 0.56*thetadot1*thetadot2*cos(theta4)*cos(theta5)*sin(theta2)*sin(theta3)*sin(theta4)*sin(theta5)*sin(theta6) + 0.56*thetadot1*thetadot3*cos(theta4)*cos(theta5)*sin(theta2)*sin(theta3)*sin(theta4)*sin(theta5)*sin(theta6) + 0.16*thetadot1^2*cos(theta2)*cos(theta3)*cos(theta4)*cos(theta5)*cos(theta6)^2*sin(theta2)*sin(theta3)*sin(theta4) + 0.16*thetadot1^2*cos(theta2)*cos(theta3)^2*cos(theta4)*cos(theta5)*cos(theta6)*sin(theta2)*sin(theta5)*sin(theta6) + 0.16*thetadot1^2*cos(theta2)^2*cos(theta3)*cos(theta4)*cos(theta5)*cos(theta6)*sin(theta3)*sin(theta5)*sin(theta6) + 0.56*thetadot1^2*cos(theta2)*cos(theta3)*cos(theta4)^2*cos(theta5)*sin(theta2)*sin(theta3)*sin(theta5)*sin(theta6) - 0.08*thetadot1*thetadot2*cos(theta2)*cos(theta3)*cos(theta4)*cos(theta5)^2*cos(theta6)*sin(theta4)*sin(theta6) - 0.08*thetadot1*thetadot3*cos(theta2)*cos(theta3)*cos(theta4)*cos(theta5)^2*cos(theta6)*sin(theta4)*sin(theta6) + 0.08*thetadot1*thetadot2*cos(theta4)*cos(theta5)^2*cos(theta6)*sin(theta2)*sin(theta3)*sin(theta4)*sin(theta6) + 0.08*thetadot1*thetadot3*cos(theta4)*cos(theta5)^2*cos(theta6)*sin(theta2)*sin(theta3)*sin(theta4)*sin(theta6) + 0.08*thetadot1^2*cos(theta2)*cos(theta3)*cos(theta4)^2*cos(theta5)^2*cos(theta6)*sin(theta2)*sin(theta3)*sin(theta6)];

 
g =[                                                                                                                                                                                                                                                                                                                                                                                                                                                                                                                                                                                                                                                                                                                                                                                                                                                                                                                                                                                                                                                       0;
24.525*sin(theta2)*sin(theta3) - 1.962*sin(theta2) - 24.525*cos(theta2)*cos(theta3) - 1.962*cos(theta2)*sin(theta3) - 1.962*cos(theta3)*sin(theta2) - 23.544*cos(theta2) - 27.468*cos(theta5)*sin(theta2)*sin(theta3) + 1.962*sin(theta2)*sin(theta3)*sin(theta5) + 27.468*cos(theta2)*cos(theta3)*cos(theta5) - 1.962*cos(theta2)*cos(theta4)*sin(theta3) - 1.962*cos(theta3)*cos(theta4)*sin(theta2) - 1.962*cos(theta2)*cos(theta3)*sin(theta5) - 1.962*cos(theta2)*cos(theta4)*cos(theta5)*sin(theta3) - 1.962*cos(theta3)*cos(theta4)*cos(theta5)*sin(theta2) - 1.962*cos(theta2)*cos(theta3)*cos(theta6)*sin(theta5) - 27.468*cos(theta2)*cos(theta4)*sin(theta3)*sin(theta5) - 27.468*cos(theta3)*cos(theta4)*sin(theta2)*sin(theta5) + 1.962*cos(theta2)*sin(theta3)*sin(theta4)*sin(theta6) + 1.962*cos(theta3)*sin(theta2)*sin(theta4)*sin(theta6) + 1.962*cos(theta6)*sin(theta2)*sin(theta3)*sin(theta5) - 1.962*cos(theta2)*cos(theta4)*cos(theta5)*cos(theta6)*sin(theta3) - 1.962*cos(theta3)*cos(theta4)*cos(theta5)*cos(theta6)*sin(theta2);
                                         24.525*sin(theta2)*sin(theta3) - 1.962*cos(theta2)*sin(theta3) - 1.962*cos(theta3)*sin(theta2) - 24.525*cos(theta2)*cos(theta3) - 27.468*cos(theta5)*sin(theta2)*sin(theta3) + 1.962*sin(theta2)*sin(theta3)*sin(theta5) + 27.468*cos(theta2)*cos(theta3)*cos(theta5) - 1.962*cos(theta2)*cos(theta4)*sin(theta3) - 1.962*cos(theta3)*cos(theta4)*sin(theta2) - 1.962*cos(theta2)*cos(theta3)*sin(theta5) - 1.962*cos(theta2)*cos(theta4)*cos(theta5)*sin(theta3) - 1.962*cos(theta3)*cos(theta4)*cos(theta5)*sin(theta2) - 1.962*cos(theta2)*cos(theta3)*cos(theta6)*sin(theta5) - 27.468*cos(theta2)*cos(theta4)*sin(theta3)*sin(theta5) - 27.468*cos(theta3)*cos(theta4)*sin(theta2)*sin(theta5) + 1.962*cos(theta2)*sin(theta3)*sin(theta4)*sin(theta6) + 1.962*cos(theta3)*sin(theta2)*sin(theta4)*sin(theta6) + 1.962*cos(theta6)*sin(theta2)*sin(theta3)*sin(theta5) - 1.962*cos(theta2)*cos(theta4)*cos(theta5)*cos(theta6)*sin(theta3) - 1.962*cos(theta3)*cos(theta4)*cos(theta5)*cos(theta6)*sin(theta2);
                                                                                                                                                                                                                                                                                                                                                                                                                                                                                                                                                                                                                                                                                                                                                                                                                                                                                      -(981*cos(theta2 + theta3)*(sin(theta4) + cos(theta5)*sin(theta4) + cos(theta4)*sin(theta6) + 14.0*sin(theta4)*sin(theta5) + cos(theta5)*cos(theta6)*sin(theta4)))/500;
                                                                                                                                                                                                                                                                                                                                                                                   27.468*cos(theta2)*cos(theta3)*cos(theta4)*cos(theta5) - 27.468*cos(theta3)*sin(theta2)*sin(theta5) - 1.962*cos(theta2)*cos(theta5)*sin(theta3) - 1.962*cos(theta3)*cos(theta5)*sin(theta2) - 27.468*cos(theta2)*sin(theta3)*sin(theta5) - 1.962*cos(theta2)*cos(theta3)*cos(theta4)*sin(theta5) - 1.962*cos(theta2)*cos(theta5)*cos(theta6)*sin(theta3) - 1.962*cos(theta3)*cos(theta5)*cos(theta6)*sin(theta2) - 27.468*cos(theta4)*cos(theta5)*sin(theta2)*sin(theta3) + 1.962*cos(theta4)*sin(theta2)*sin(theta3)*sin(theta5) - 1.962*cos(theta2)*cos(theta3)*cos(theta4)*cos(theta6)*sin(theta5) + 1.962*cos(theta4)*cos(theta6)*sin(theta2)*sin(theta3)*sin(theta5);
                                                                                                                                                                                                                                                                                                                                                                                                                                                                                                                                                                                                                                                                                       1.962*cos(theta6)*sin(theta2)*sin(theta3)*sin(theta4) - 1.962*cos(theta2)*cos(theta3)*cos(theta6)*sin(theta4) + 1.962*cos(theta2)*sin(theta3)*sin(theta5)*sin(theta6) + 1.962*cos(theta3)*sin(theta2)*sin(theta5)*sin(theta6) - 1.962*cos(theta2)*cos(theta3)*cos(theta4)*cos(theta5)*sin(theta6) + 1.962*cos(theta4)*cos(theta5)*sin(theta2)*sin(theta3)*sin(theta6)];

Fr=[2*thetadot1+2*sign(thetadot1);
    2*thetadot2+2*sign(thetadot2);
    5*thetadot3+5*sign(thetadot3);
    5*thetadot4+5*sign(thetadot4);
    5*thetadot5+5*sign(thetadot5);
    5*thetadot6+5*sign(thetadot6)];

% Fr=[2.1*thetadot1+2*sign(thetadot1);
%     3*thetadot2+2*sign(thetadot2);
%     2.5*thetadot3+1.5*sign(thetadot3);
%     zeros(3,1)];
disturb=[7*sin(thetadot1);
    6*sin(thetadot2);
    4*sin(thetadot3);
    2*sin(thetadot4);
    5*sin(thetadot5);
    5*sin(thetadot6)];
% disturb=[7.2*sin(thetadot1);
%     6.1*sin(thetadot2);
%     4.5*sin(thetadot3);
%     zeros(3,1)];

x=[theta;thetadot];
dx=zeros(12,1);
dx(1)=x(7);
dx(2)=x(8);
dx(3)=x(9);
dx(4)=x(10);
dx(5)=x(11);
dx(6)=x(12);

dx(7:12)=inv(MM)*(u-C-g-Fr-disturb);
disturbance=inv(MM)*(-Fr-disturb);
y=[dx(1);dx(2);dx(3);dx(4);dx(5);dx(6);dx(7);dx(8);dx(9);dx(10);dx(11);dx(12)];
